simulink model "lqr_finito_nivel_matlab2015b"  (R2015b)
settings: Solver=ode15s  StartTime=0.0  StopTime=30  RelTol=1e-3
values from neighbouring files (symbols this model uses):
  A = [-0.1107 0;0.1107 -0.1107]    [ejecutar_solucion_nivel.m]
  B = [-1 1;0 0]    [ejecutar_solucion_nivel.m]
  R = 100*[1 0;0 0.1]    [ejecutar_solucion_nivel.m]
settings Model: Creator=Juan Pablo Requez  LastModifiedBy=Juan Pablo Requez
settings DataIOCC: LimitDataPoints=off
settings DebuggingCC: AllowSymbolicDim=on
settings ModelReferenceCC: PropagateSignalLabelsOutOfModel=on
settings GRTTargetCC: GeneratePreprocessorConditionals=Disable all

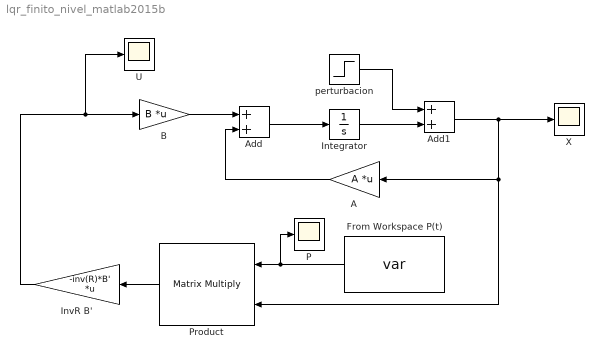
== system lqr_finito_nivel_matlab2015b ==
  A : Gain  Gain=A  Multiplication=Matrix(K*u)
  Add : Sum
  Add1 : Sum
  B : Gain  Gain=B  Multiplication=Matrix(K*u)
  From Workspace P(t) : FromWorkspace  VariableName=var  SampleTime=0  OutputAfterFinalValue=Setting to zero
  Integrator : Integrator  InitialCondition=[0.1 0.1]
  InvR B' : Gain  Gain=-inv(R)*B'  Multiplication=Matrix(K*u)
  P : Scope
  Product : Product  Multiplication=Matrix(*)
  U : Scope
  X : Scope
  perturbacion : Step  Time=0  After=0  SampleTime=0
  wires:
  B/1 -> Add/1
  Add/1 -> Integrator/1
  InvR B'/1 -> U/1, B/1
  perturbacion/1 -> Add1/1
  Product/1 -> InvR B'/1
  A/1 -> Add/2
  Add1/1 -> X/1, Product/2, A/1
  Integrator/1 -> Add1/2
  From Workspace P(t)/1 -> P/1, Product/1
